simulink model "Tesla_ModY_andalib_updated_batt_sizing"  (R2023a)
settings: Solver=VariableStepAuto  StartTime=0.0  StopTime=240  RelTol=1e-9
values from neighbouring files (symbols this model uses):
  gross_weight_kg = 1232 + calculated_bat_weight    (= 2003.0014)    [bat_cal.m]
libraries: slpidlib x2, simulink_extras x1, autolibdatasheetbattery x1, simulink x1
settings Model: Creator=ASUS  LastModifiedBy=ASUS

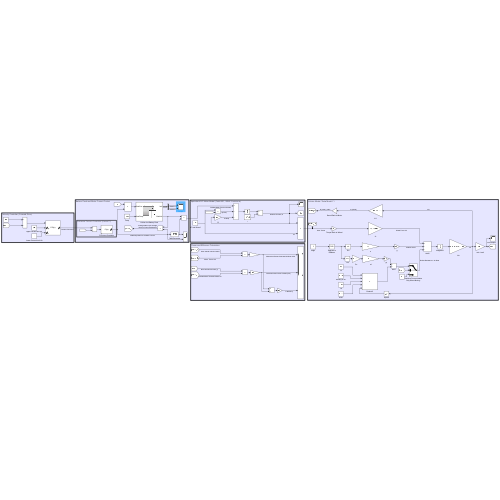
[thumbnail: Simulink's stored preview of the top-level diagram]
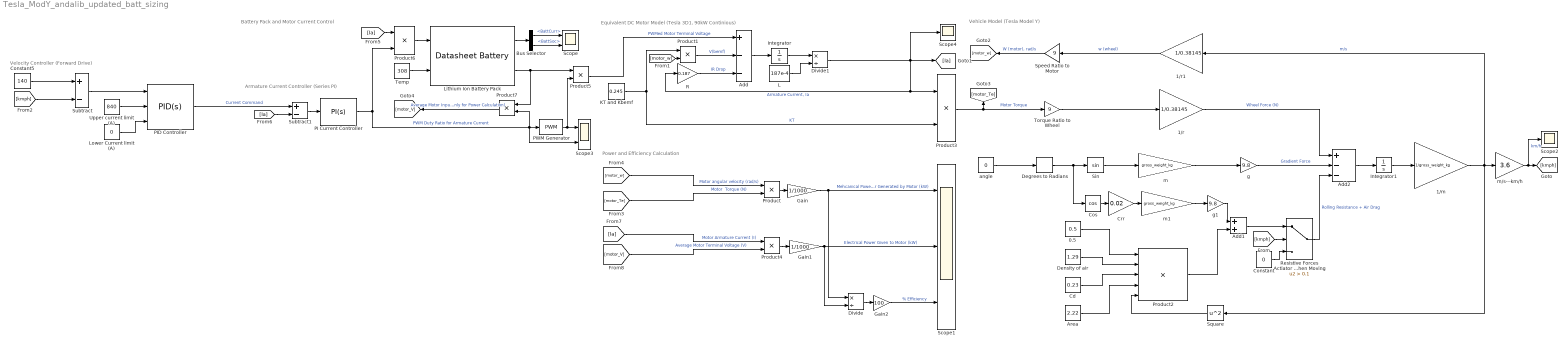
== system Tesla_ModY_andalib_updated_batt_sizing ==
  note: Power and Efficiency Calculation
  note: Velocity Controller (Forward Drive)
  note: Armature Current Controller (Series PI)
  note: Battery Pack and Motor Current Control
  note: Equivalent DC Motor Model (Tesla 3D1, 90kW Continious)
  note: Vehicle Model (Tesla Model Y)
  0.5 : Constant  Value=0.5
  1/m : Gain  Gain=1/gross_weight_kg
  1/r : Gain  Gain=1/0.38145
  1/r1 : Gain  Gain=1/0.38145
  Add : Sum  Inputs=+--
  Add1 : Sum
  Add2 : Sum  Inputs=+--
  Area : Constant  Value=2.22
  Bus Selector : BusSelector  OutputSignals=BattCurr,BattSoc
  Cd : Constant  Value=0.23
  Constant : Constant  Value=0
  Constant5 : Constant  Value=140
  Cos : Trigonometry  Operator=cos
  Crr : Gain  Gain=0.02
  Degrees to Radians : simulink_extras/Transformations/Degrees to Radians
  Density of air : Constant  Value=1.29
  Divide : Product  Inputs=*/
  Divide1 : Product  Inputs=*/
  Gain : Gain  Gain=1/1000
  Gain1 : Gain  Gain=1/1000
  Gain2 : Gain  Gain=100
  Integrator : Integrator
  Integrator1 : Integrator
  KT and Kbemf : Constant  Value=0.245
  L : Constant  Value=187e-4
  Lithium Ion Battery Pack : autolibdatasheetbattery/Datasheet Battery  CapacityCtrl=Parameter  OutputVlt=Unfiltered  BattChargeMax=cell_cap_Ah  Em=[2.8 3.228 3.284 3.361 3.408 3.427 3.472 3.477 3.493 3.504 3.516 3.528 3.537 3.545 3.555 3.561 3.566 3.576 3.587 3.589 3.594 3.6 3.608 3.61 3.616 3.619 3.626 3.632 3.637 3.64 3.645 3.646 3.652 3.655 3.658 3.661 3.664 3.668 3.673 3.678 3.68 3.681 3.686 3.692 3.699 3.702 3.705 3.71 3.717 3.723 3.728 3.733 3.735 3.742 3.749 3.755 3.761 3.768 3.773 3.78 3.791 3.798 3.798 3.814 3.818 3.825 3.841 3.846 3.855 3.863 3.877 3.885 3.894 3.907 3.919 3.926 3.935 3.944 3.954 3.964 3.974 3.988 3.998 4.014 4.029 4.034 4.047 4.065 4.074 4.086 4.097 4.131 4.126 4.138 4.15 4.18 4.174 4.187 4.207 4.231 4.221]  CapLUTBp=[0 0.01 0.02 0.03 0.04 0.05 0.06 0.07 0.08 0.09 0.1 0.11 0.12 0.13 0.14 0.15 0.16 0.17 0.18 0.19 0.2 0.21 0.22 0.23 0.24 0.25 0.26 0.27 0.28 0.29 0.3 0.31 0.32 0.33 0.34 0.35 0.36 0.37 0.38 0.39 0.4 0.41 0.42 0.43 0.44 0.45 0.46 0.47 0.48 0.49 0.5 0.51 0.52 0.53 0.54 0.55 0.56 0.57 0.58 0.59 0.6 0.61 0.62 0.63 0.64 0.65 0.66 0.67 0.68 0.69 0.7 0.71 0.72 0.73 0.74 0.75 0.76 0.77 0.78 0.79 0.8 0.81 0.82 0.83 0.84 0.85 0.86 0.87 0.88 0.89 0.9 0.91 0.92 0.93 0.94 0.95 0.96 0.97 0.98 0.99 1]  RInt=[0.008846 0.009319 0.009027 0.00847 0.01032 0.01314;0.006389 0.006554 0.005553 0.005525 0.006043 0.007805;0.004364 0.004101 0.00406 0.003452 0.003846 0.004517;0.002031 0.002563 0.002532 0.00246 0.002716 0.003047;0.001443 0.001825 0.001795 0.001778 0.001924 0.002234;0.0005603 0.0007192 0.0006887 0.0007557 0.0007355 0.001014;0.001028 0.001338 0.001 0.001536 0.001546 0.002789]  BattTempBp=[243.1 253.1 263.1 273.1 283.1 298.1 313.1]  CapSOCBp=[0 0.2 0.4 0.6 0.8 1]  Ns=96  Np=no_cells_parallel  BattCapInit=4.8  Tc=1/1000  Vinit=3.75*72  RefBlkName='autolibdatasheetbattery/Datasheet Battery'
  Lower Current limit (A) : Constant  Value=0
  PI Current Controller : slpidlib/PID Controller  Controller=PI  Form=Ideal  TimeDomain=Continuous-time  UseExternalTs=off  SampleTime=-1  IntegratorMethod=Forward Euler  FilterMethod=Forward Euler  ControllerParametersSource=internal  P=0.001  I=11.75  UseKiTs=off  D=0  N=100  UseFilter=on  TunerSelectOption=Transfer Function Based (PID Tuner App)  InitialConditionSource=internal  InitialConditionForIntegrator=0  InitialConditionForFilter=0  DifferentiatorICPrevScaledInput=0  ExternalReset=none  TrackingMode=off  Kt=1  LimitOutput=on  SatLimitsSource=internal  UpperSaturationLimit=1  LowerSaturationLimit=0  LinearizeAsGain=on  AntiWindupMode=clamping  Kb=1  LimitIntegrator=off  UpperIntegratorSaturationLimit=inf  LowerIntegratorSaturationLimit=-inf  RndMeth=Convergent  POutMin=[]  POutMax=[]  IOutMin=[]  IOutMax=[]  DOutMin=[]  DOutMax=[]  NOutMin=[]  NOutMax=[]  SumOutMin=[]  SumOutMax=[]  SaturationOutMin=[]  SaturationOutMax=[]  PParamMin=[]  PParamMax=[]  IParamMin=[]  IParamMax=[]  DParamMin=[]  DParamMax=[]  NParamMin=[]  NParamMax=[]  KbParamMin=[]  KbParamMax=[]  KtParamMin=[]  KtParamMax=[]  KbOutMin=[]  KbOutMax=[]  KtOutMin=[]  KtOutMax=[]  IntegratorOutMin=[]  IntegratorOutMax=[]  FilterOutMin=[]  FilterOutMax=[]  SumI1OutMin=[]  SumI1OutMax=[]  SumI2OutMin=[]  SumI2OutMax=[]  SumI3OutMin=[]  SumI3OutMax=[]  SumI4OutMin=[]  SumI4OutMax=[]  SumDOutMin=[]  SumDOutMax=[]  DifferentiatorOutMin=[]  DifferentiatorOutMax=[]  FilterDiffOutCoefMin=[]  FilterDiffOutCoefMax=[]  ReciprocalOutMin=[]  ReciprocalOutMax=[]  SumDenOutMin=[]  SumDenOutMax=[]  SumNumOutMin=[]  SumNumOutMax=[]  DivideOutMin=[]  DivideOutMax=[]  UdiffTsProdOutMin=[]  UdiffTsProdOutMax=[]  NTsProdOutMin=[]  NTsProdOutMax=[]  UintegralTsProdOutMin=[]  UintegralTsProdOutMax=[]  UngainTsProdOutMin=[]  UngainTsProdOutMax=[]  ClampingZeroOutDataTypeStr=Inherit: Inherit via back propagation  ClampingZeroOutMin=[]  ClampingZeroOutMax=[]  FilterDenConstantOutDataTypeStr=Inherit: Inherit via back propagation  FilterDenConstantOutMin=[]  FilterDenConstantOutMax=[]  PCopyOutDataTypeStr=Inherit: Inherit via back propagation  PCopyOutMin=[]  PCopyOutMax=[]  NCopyOutDataTypeStr=Inherit: Inherit via back propagation  NCopyOutMin=[]  NCopyOutMax=[]  IntegratorContinuousStateAttributes=''  IntegratorStateMustResolveToSignalObject=off  IntegratorRTWStateStorageClass=Auto  FilterContinuousStateAttributes=''  FilterStateMustResolveToSignalObject=off  FilterRTWStateStorageClass=Auto  ParallelPVariant=Passthrough  IdealPVariant=InternalParameters  IVariant=InternalParameters  DVariant=Disabled  IntegratorVariant=Continuous  SatVariant=Enabled  AWVariant=ContClampingIdeal  PCopyVariant=InternalParamsIdeal  TRVariant=Disabled  FdbkBlocksVariant=Forward  IdealPFdbkVariant=Disabled  SatFdbkVariant=Disabled  DerivativeFilterVariant=Disabled  NVariant=Disabled  NCopyVariant=Disabled_SignalSpec  FilterICVariant=Disabled  IntegratorICVariant=InternalICs  ExternalResetVariant=Disabled  TRSumVariant=Passthrough  SumFdbkVariant=Disabled  SumVariant=Sum_PI  TsampFilterVariant=InternalTs  TsampNgainVariant=Passthrough  TsampIntegralVariant=Disabled_SignalSpec  ExternalSaturationOutDataTypeStr=Inherit: Same as second input
  PID Controller : slpidlib/PID Controller  Controller=PID  Form=Parallel  TimeDomain=Continuous-time  UseExternalTs=off  SampleTime=-1  IntegratorMethod=Forward Euler  FilterMethod=Forward Euler  ControllerParametersSource=internal  P=100  I=10  UseKiTs=off  D=0  N=100  UseFilter=on  TunerSelectOption=Transfer Function Based (PID Tuner App)  InitialConditionSource=internal  InitialConditionForIntegrator=0  InitialConditionForFilter=0  DifferentiatorICPrevScaledInput=0  ExternalReset=none  TrackingMode=off  Kt=1  LimitOutput=on  SatLimitsSource=external  UpperSaturationLimit=1  LowerSaturationLimit=0  LinearizeAsGain=off  AntiWindupMode=clamping  Kb=1  LimitIntegrator=off  UpperIntegratorSaturationLimit=inf  LowerIntegratorSaturationLimit=-inf  POutMin=[]  POutMax=[]  IOutMin=[]  IOutMax=[]  DOutMin=[]  DOutMax=[]  NOutMin=[]  NOutMax=[]  SumOutMin=[]  SumOutMax=[]  SaturationOutMin=[]  SaturationOutMax=[]  PParamMin=[]  PParamMax=[]  IParamMin=[]  IParamMax=[]  DParamMin=[]  DParamMax=[]  NParamMin=[]  NParamMax=[]  KbParamMin=[]  KbParamMax=[]  KtParamMin=[]  KtParamMax=[]  KbOutMin=[]  KbOutMax=[]  KtOutMin=[]  KtOutMax=[]  IntegratorOutMin=[]  IntegratorOutMax=[]  FilterOutMin=[]  FilterOutMax=[]  SumI1OutMin=[]  SumI1OutMax=[]  SumI2OutMin=[]  SumI2OutMax=[]  SumI3OutMin=[]  SumI3OutMax=[]  SumI4OutMin=[]  SumI4OutMax=[]  SumDOutMin=[]  SumDOutMax=[]  DifferentiatorOutMin=[]  DifferentiatorOutMax=[]  FilterDiffOutCoefMin=[]  FilterDiffOutCoefMax=[]  ReciprocalOutMin=[]  ReciprocalOutMax=[]  SumDenOutMin=[]  SumDenOutMax=[]  SumNumOutMin=[]  SumNumOutMax=[]  DivideOutMin=[]  DivideOutMax=[]  UdiffTsProdOutMin=[]  UdiffTsProdOutMax=[]  NTsProdOutMin=[]  NTsProdOutMax=[]  UintegralTsProdOutMin=[]  UintegralTsProdOutMax=[]  UngainTsProdOutMin=[]  UngainTsProdOutMax=[]  ClampingZeroOutDataTypeStr=Inherit: Inherit via back propagation  ClampingZeroOutMin=[]  ClampingZeroOutMax=[]  FilterDenConstantOutDataTypeStr=Inherit: Inherit via back propagation  FilterDenConstantOutMin=[]  FilterDenConstantOutMax=[]  PCopyOutDataTypeStr=Inherit: Inherit via back propagation  PCopyOutMin=[]  PCopyOutMax=[]  NCopyOutDataTypeStr=Inherit: Inherit via back propagation  NCopyOutMin=[]  NCopyOutMax=[]  IntegratorContinuousStateAttributes=''  IntegratorStateMustResolveToSignalObject=off  IntegratorRTWStateStorageClass=Auto  FilterContinuousStateAttributes=''  FilterStateMustResolveToSignalObject=off  FilterRTWStateStorageClass=Auto  ParallelPVariant=InternalParameters  IdealPVariant=Disabled  IVariant=InternalParameters  DVariant=InternalParameters  IntegratorVariant=Continuous  SatVariant=External  AWVariant=ContClampingParallel  PCopyVariant=Disabled  TRVariant=Disabled  FdbkBlocksVariant=Forward  IdealPFdbkVariant=Disabled  SatFdbkVariant=Disabled  DerivativeFilterVariant=ContFilter  NVariant=InternalParameters  NCopyVariant=Disabled  FilterICVariant=InternalICsFilter  IntegratorICVariant=InternalICs  ExternalResetVariant=Disabled  TRSumVariant=Passthrough  SumFdbkVariant=Disabled  SumVariant=Sum_PID  TsampFilterVariant=InternalTs  TsampNgainVariant=Passthrough  TsampIntegralVariant=Disabled_SignalSpec  ExternalSaturationOutDataTypeStr=Inherit: Same as second input
  PWM Generator : simulink/Discontinuities/PWM  DisableCoverage=on  Period=1e-4  InitialDelay=0  DisallowZeroDutyCycle=off  RunAtFixedTimeIntervals=off  SampleTime=0.1
  Product{,1,3..7} (7 alike) : Product
  Product2 : Product  Inputs=5
  R : Gain  Gain=0.187
  "Resistive Forces Actiator Only When Moving " : Switch  Criteria=u2 > Threshold  Threshold=0.1  SaturateOnIntegerOverflow=off  InputSameDT=off
  Scope : Scope  NumInputPorts=2
  Scope1 : Scope  NumInputPorts=3
  Scope2 : Scope
  Scope3 : Scope  NumInputPorts=2
  Scope4 : Scope
  Sin : Trigonometry
  Speed Ratio to Motor : Gain  Gain=9
  Square : Math  Operator=square
  Subtract : Sum  Inputs=+-
  Subtract1 : Sum  Inputs=+-
  Temp : Constant  Value=308
  Torque Ratio to Wheel : Gain  Gain=9
  Upper current limit (A) : Constant  Value=840
  angle : Constant  Value=0
  g : Gain  Gain=9.8
  g1 : Gain  Gain=9.8
  m : Gain  Gain=gross_weight_kg
  m/s---km/h : Gain  Gain=3.6
  m1 : Gain  Gain=gross_weight_kg
  wires:
  Divide1/1 -> Scope4/1, [Ia], Product3/1, R/1  "Armature Current, Ia"
  R/1 -> Add/3  "IR Drop"
  Add/1 -> Integrator/1
  KT and Kbemf/1 -> Product3/2, Product1/1  "KT"
  g/1 -> Add2/2  "Gradient Force"
  angle/1 -> Degrees to Radians/1
  1/m/1 -> m/s---km/h/1, 1/r1/1, Square/1  "m/s"
  Integrator1/1 -> 1/m/1
  Density of air/1 -> Product2/2
  0.5/1 -> Product2/1
  Degrees to Radians/1 -> Sin/1, Cos/1
  Cd/1 -> Product2/3
  Area/1 -> Product2/4
  Square/1 -> Product2/5
  m/s---km/h/1 -> [kmph], Scope2/1  "km/h"
  Cos/1 -> Crr/1
  Torque Ratio to Wheel/1 -> 1/r/1
  1/r/1 -> Add2/1  "Wheel Force (N)"
  Add2/1 -> Integrator1/1
  Product3/1 -> Torque Ratio to Wheel/1, [motor_Te]  "Motor Torque"
  1/r1/1 -> Speed Ratio to Motor/1  "w (wheel)"
  Subtract/1 -> PID Controller/1
  Constant5/1 -> Subtract/1
  Subtract1/1 -> PI Current Controller/1
  Lower Current limit (A)/1 -> PID Controller/3
  Upper current limit (A)/1 -> PID Controller/2
  Sin/1 -> m/1
  m/1 -> g/1
  Crr/1 -> m1/1
  m1/1 -> g1/1
  g1/1 -> Add1/1
  Product2/1 -> Add1/2
  "Resistive Forces Actiator Only When Moving "/1 -> Add2/3  "Rolling Resistance + Air Drag"
  [kmph] -> "Resistive Forces Actiator Only When Moving "/2
  Add1/1 -> "Resistive Forces Actiator Only When Moving "/1
  Constant/1 -> "Resistive Forces Actiator Only When Moving "/3
  Speed Ratio to Motor/1 -> [motor_w]  "W (motor), rad/s"
  [motor_w] -> Product1/2
  Temp/1 -> Lithium Ion Battery Pack/2
  PI Current Controller/1 -> Product6/2, Scope3/2, PWM Generator/1, Product7/2  "PWM Duty Ratio for Armature Current"
  [Ia] -> Product6/1
  [Ia] -> Subtract1/2
  Lithium Ion Battery Pack/1 -> Bus Selector/1
  Bus Selector/1 -> Scope/1  "<BattCurr>"
  Bus Selector/2 -> Scope/2  "<BattSoc>"
  PID Controller/1 -> Subtract1/1  "Current Command"
  Product1/1 -> Add/2  "V(bemf)"
  [kmph] -> Subtract/2
  L/1 -> Divide1/2
  Integrator/1 -> Divide1/1
  Product6/1 -> Lithium Ion Battery Pack/1
  Lithium Ion Battery Pack/2 -> Product5/1, Product7/1
  Product5/1 -> Add/1  "PWMed Motor Terminal Voltage"
  PWM Generator/1 -> Product5/2, Scope3/1
  [motor_w] -> Product/1  "Motor angular velocity (rad/s)"
  [motor_Te] -> Product/2  "Motor  Torque (N)"
  Product/1 -> Gain/1
  Gain/1 -> Scope1/1, Divide/1  "Mehcanical Power Generated by Motor (kW)"
  [Ia] -> Product4/1  "Motor Armature Current (I)"
  [motor_V] -> Product4/2  "Average Motor Terminal Voltage (V)"
  Product4/1 -> Gain1/1
  Gain1/1 -> Scope1/2, Divide/2  "Electrical Power Given to Motor (kW)"
  Divide/1 -> Gain2/1
  Gain2/1 -> Scope1/3  "% Efficiency"
  Product7/1 -> [motor_V]  "Average Motor Input Voltage (Only for Power Calculation)"
